simulink model "traj"  (R2020b)
settings: Solver=VariableStepAuto  StartTime=0.0  StopTime=All_Sim_time  MaxStep=0.05  RelTol=1e-3
model workspace (MAT data in the model file):
  Delay = 1
undefined symbols (not defined in the file or in its folder): All_Delay_betwn_actns, All_Maneuver_smoothness, Maneuver1_aggression, Maneuver2_aggression, Maneuver3_aggression, Maneuver4_aggression, Maneuver5_aggression
settings Model: Creator=pyoty  LastModifiedBy=liors

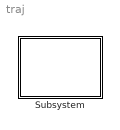
== system traj ==
  Subsystem : Subsystem

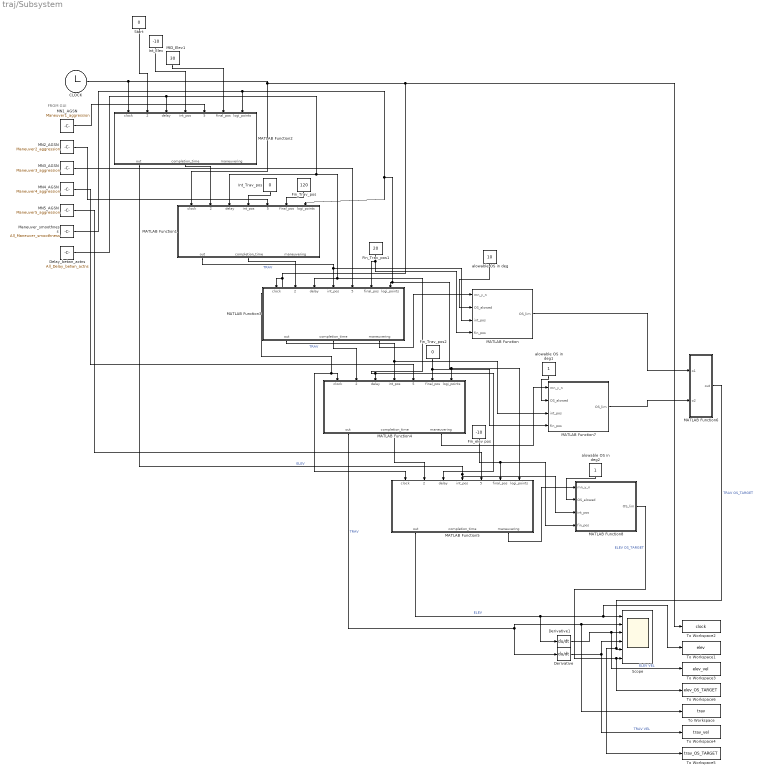
== system traj/Subsystem ==
  note: FROM GUI
  CLOCK : Clock
  Delay_betwn_actns : Constant  Value=All_Delay_betwn_actns
  Derivative : Derivative
  Derivative1 : Derivative
  Fin_Trav_pos : Constant  Value=120
  Fin_Trav_pos1 : Constant  Value=20
  Fin_Trav_pos2 : Constant  Value=0
  Fin_elev pos : Constant  Value=-10
  Int_Elev : Constant  Value=-10
  Int_Trav_pos : Constant  Value=0
  MATLAB Function : MATLAB Function  TreatAsAtomicUnit=on
  MATLAB Function1 : MATLAB Function  TreatAsAtomicUnit=on
  MATLAB Function2 : MATLAB Function  TreatAsAtomicUnit=on
  MATLAB Function3 : MATLAB Function  TreatAsAtomicUnit=on
  MATLAB Function4 : MATLAB Function  TreatAsAtomicUnit=on
  MATLAB Function5 : MATLAB Function  TreatAsAtomicUnit=on
  MATLAB Function6 : MATLAB Function  TreatAsAtomicUnit=on
  MATLAB Function7 : MATLAB Function  TreatAsAtomicUnit=on
  MATLAB Function8 : MATLAB Function  TreatAsAtomicUnit=on
  MID_Elev1 : Constant  Value=30
  MN1_AGSN : Constant  Value=Maneuver1_aggression
  MN2_AGSN : Constant  Value=Maneuver2_aggression
  MN3_AGSN : Constant  Value=Maneuver3_aggression
  MN4_AGSN : Constant  Value=Maneuver4_aggression
  MN5_AGSN : Constant  Value=Maneuver5_aggression
  Maneuver_smoothness : Constant  Value=All_Maneuver_smoothness
  Scope : Scope  NumInputPorts=6
  Start : Constant  Value=0
  To Workspace : ToWorkspace  VariableName=trav  SaveFormat=Timeseries  SampleTime=-1
  To Workspace1 : ToWorkspace  VariableName=elev  SaveFormat=Timeseries  SampleTime=-1
  To Workspace2 : ToWorkspace  VariableName=clock  SaveFormat=Timeseries  SampleTime=-1
  To Workspace3 : ToWorkspace  VariableName=elev_vel  SaveFormat=Timeseries  SampleTime=-1
  To Workspace4 : ToWorkspace  VariableName=trav_vel  SaveFormat=Timeseries  SampleTime=-1
  To Workspace5 : ToWorkspace  VariableName=trav_OS_TARGET  SaveFormat=Timeseries  SampleTime=-1
  To Workspace6 : ToWorkspace  VariableName=elev_OS_TARGET  SaveFormat=Timeseries  SampleTime=-1
  alowable OS in deg : Constant  Value=10
  alowable OS in deg1 : Constant
  alowable OS in deg2 : Constant
  wires:
  Derivative1/1 -> To Workspace3/1, Scope/3  "ELEV VEL"
  CLOCK/1 -> To Workspace2/1, MATLAB Function4/1(clock), MATLAB Function5/1(clock), MATLAB Function3/1(clock), MATLAB Function1/1(clock), MATLAB Function2/1(clock)
  MATLAB Function3/3(maneuvering) -> MATLAB Function/1(mn_y_n)
  Fin_elev pos/1 -> MATLAB Function8/4(fin_pos), MATLAB Function5/6(final_pos)
  MATLAB Function2/1(out) -> MATLAB Function8/3(int_pos), MATLAB Function5/4(int_pos)  "ELEV"
  Maneuver_smoothness/1 -> MATLAB Function4/7(logi_points), MATLAB Function5/7(logi_points), MATLAB Function3/7(logi_points), MATLAB Function1/7(logi_points), MATLAB Function2/7(logi_points)
  Int_Elev/1 -> MATLAB Function2/4(int_pos)
  Derivative/1 -> Scope/4, To Workspace4/1  "TRAV VEL"
  Start/1 -> MATLAB Function2/2(pev_mn_fin_time)
  MATLAB Function7/1(OS_lim) -> MATLAB Function6/2(o2)
  MN2_AGSN/1 -> MATLAB Function1/5(agressivness)
  MATLAB Function5/1(out) -> To Workspace1/1, Scope/1, Derivative1/1  "ELEV"
  MATLAB Function3/1(out) -> MATLAB Function7/3(int_pos), MATLAB Function4/4(int_pos)  "TRAV"
  alowable OS in deg1/1 -> MATLAB Function7/2(OS_alowed)
  Fin_Trav_pos1/1 -> MATLAB Function/4(fin_pos), MATLAB Function3/6(final_pos)
  MN5_AGSN/1 -> MATLAB Function5/5(agressivness)
  MATLAB Function1/1(out) -> MATLAB Function/3(int_pos), MATLAB Function3/4(int_pos)  "TRAV"
  Delay_betwn_actns/1 -> MATLAB Function5/3(delay), MATLAB Function4/3(delay), MATLAB Function3/3(delay), MATLAB Function1/3(delay), MATLAB Function2/3(delay)
  MN4_AGSN/1 -> MATLAB Function4/5(agressivness)
  MN1_AGSN/1 -> MATLAB Function2/5(agressivness)
  Int_Trav_pos/1 -> MATLAB Function1/4(int_pos)
  MATLAB Function3/2(completion_time) -> MATLAB Function4/2(pev_mn_fin_time)
  Fin_Trav_pos2/1 -> MATLAB Function7/4(fin_pos), MATLAB Function4/6(final_pos)
  alowable OS in deg/1 -> MATLAB Function/2(OS_alowed)
  MATLAB Function1/2(completion_time) -> MATLAB Function3/2(pev_mn_fin_time)
  MATLAB Function5/3(maneuvering) -> MATLAB Function8/1(mn_y_n)
  MATLAB Function2/2(completion_time) -> MATLAB Function1/2(pev_mn_fin_time)
  MN3_AGSN/1 -> MATLAB Function3/5(agressivness)
  Fin_Trav_pos/1 -> MATLAB Function1/6(final_pos)
  MID_Elev1/1 -> MATLAB Function2/6(final_pos)
  MATLAB Function4/1(out) -> Derivative/1, To Workspace/1, Scope/2  "TRAV"
  MATLAB Function6/1(out) -> To Workspace5/1, Scope/5  "TRAV OS_TARGET"
  MATLAB Function8/1(OS_lim) -> To Workspace6/1, Scope/6  "ELEV OS_TARGET"
  alowable OS in deg2/1 -> MATLAB Function8/2(OS_alowed)
  MATLAB Function/1(OS_lim) -> MATLAB Function6/1(o1)
  MATLAB Function4/3(maneuvering) -> MATLAB Function7/1(mn_y_n)
  MATLAB Function4/2(completion_time) -> MATLAB Function5/2(pev_mn_fin_time)

== matlab function traj/Subsystem/MATLAB Function ==
  data: mn_y_n input; OS_lim output; OS_alowed input; int_pos input; fin_pos input
function OS_lim = OS(mn_y_n,OS_alowed,int_pos,fin_pos)
if fin_pos>int_pos
    direction=1
else
    direction=-1
end

OS_lim = mn_y_n*(fin_pos+OS_alowed*direction);
if OS_lim==-inf
   OS_lim=inf
end
end

== matlab function traj/Subsystem/MATLAB Function6 ==
  data: o1 input; out output; o2 input
function out= min(o1,o2)
out=min([o1,o2])
end

== matlab function traj/Subsystem/MATLAB Function7 ==
  data: mn_y_n input; OS_lim output; OS_alowed input; int_pos input; fin_pos input
function OS_lim = OS(mn_y_n,OS_alowed,int_pos,fin_pos)
if fin_pos>int_pos
    direction=1
else
    direction=-1
end

OS_lim = mn_y_n*(fin_pos+OS_alowed*direction);
if OS_lim==-inf
   OS_lim=inf
end
end

== matlab function traj/Subsystem/MATLAB Function8 ==
  data: mn_y_n input; OS_lim output; OS_alowed input; int_pos input; fin_pos input
function OS_lim = OS(mn_y_n,OS_alowed,int_pos,fin_pos)
if fin_pos>int_pos
    direction=1
else
    direction=-1
end

OS_lim = mn_y_n*(fin_pos+OS_alowed*direction);
if OS_lim==-inf
   OS_lim=inf
end
end

== matlab function traj/Subsystem/MATLAB Function1 ==
  data: clock input; pev_mn_fin_time input; delay input; int_pos input; agressivness input; final_pos input; out output; completion_time output; logi_points input; maneuvering output
function [out,completion_time,maneuvering] =maneuver(clock,pev_mn_fin_time,delay,int_pos,agressivness,final_pos,logi_points)

if final_pos>int_pos
    direction=1
else
    direction=-1
end

slope=direction*agressivness
maneuvering=inf
mn_start_time=delay+pev_mn_fin_time
mn_completion_time=(final_pos-int_pos)/slope
completion_time=mn_completion_time+mn_start_time
coarsness=mn_completion_time/(logi_points+1)
mn_clock=clock-mn_start_time
coarse_clock=coarsness*floor(mn_clock/coarsness)
mn_clock2=clock+coarsness-mn_start_time
coarse_clock2=coarsness*floor(mn_clock2/coarsness)



if mn_clock<0
    out=int_pos
elseif clock<completion_time && mn_clock>=0
    adjust=mn_completion_time/18
    out1=((slope*mn_completion_time)/(1+exp((mn_completion_time/2-coarse_clock)/adjust)))    +int_pos
    out2=((slope*mn_completion_time)/(1+exp((mn_completion_time/2-coarse_clock2)/adjust)))    +int_pos
    sawtooth=mn_clock-coarse_clock
    new_slope=(out2-out1)/(coarsness)
    out=new_slope*sawtooth+out1
else
    out=final_pos
end

if mn_clock>=mn_completion_time/2
    maneuvering=1
end

if clock>=completion_time+delay+5/mn_completion_time
         maneuvering=inf
end
end

== matlab function traj/Subsystem/MATLAB Function3 ==
  data: clock input; pev_mn_fin_time input; delay input; int_pos input; agressivness input; final_pos input; out output; completion_time output; logi_points input; maneuvering output
function [out,completion_time,maneuvering] =maneuver(clock,pev_mn_fin_time,delay,int_pos,agressivness,final_pos,logi_points)

if final_pos>int_pos
    direction=1
else
    direction=-1
end

slope=direction*agressivness
maneuvering=inf
mn_start_time=delay+pev_mn_fin_time
mn_completion_time=(final_pos-int_pos)/slope
completion_time=mn_completion_time+mn_start_time
coarsness=mn_completion_time/(logi_points+1)
mn_clock=clock-mn_start_time
coarse_clock=coarsness*floor(mn_clock/coarsness)
mn_clock2=clock+coarsness-mn_start_time
coarse_clock2=coarsness*floor(mn_clock2/coarsness)



if mn_clock<0
    out=int_pos
elseif clock<completion_time && mn_clock>=0
    adjust=mn_completion_time/18
    out1=((slope*mn_completion_time)/(1+exp((mn_completion_time/2-coarse_clock)/adjust)))    +int_pos
    out2=((slope*mn_completion_time)/(1+exp((mn_completion_time/2-coarse_clock2)/adjust)))    +int_pos
    sawtooth=mn_clock-coarse_clock
    new_slope=(out2-out1)/(coarsness)
    out=new_slope*sawtooth+out1
else
    out=final_pos
end

if mn_clock>=mn_completion_time/2
    maneuvering=1
end

if clock>=completion_time+delay+5/mn_completion_time
         maneuvering=inf
end
end

== matlab function traj/Subsystem/MATLAB Function2 ==
  data: clock input; pev_mn_fin_time input; delay input; int_pos input; agressivness input; final_pos input; out output; completion_time output; logi_points input; maneuvering output
function [out,completion_time,maneuvering] =maneuver(clock,pev_mn_fin_time,delay,int_pos,agressivness,final_pos,logi_points)

if final_pos>int_pos
    direction=1
else
    direction=-1
end

slope=direction*agressivness
maneuvering=inf
mn_start_time=delay+pev_mn_fin_time
mn_completion_time=(final_pos-int_pos)/slope
completion_time=mn_completion_time+mn_start_time
coarsness=mn_completion_time/(logi_points+1)
mn_clock=clock-mn_start_time
coarse_clock=coarsness*floor(mn_clock/coarsness)
mn_clock2=clock+coarsness-mn_start_time
coarse_clock2=coarsness*floor(mn_clock2/coarsness)



if mn_clock<0
    out=int_pos
elseif clock<completion_time && mn_clock>=0
    adjust=mn_completion_time/18
    out1=((slope*mn_completion_time)/(1+exp((mn_completion_time/2-coarse_clock)/adjust)))    +int_pos
    out2=((slope*mn_completion_time)/(1+exp((mn_completion_time/2-coarse_clock2)/adjust)))    +int_pos
    sawtooth=mn_clock-coarse_clock
    new_slope=(out2-out1)/(coarsness)
    out=new_slope*sawtooth+out1
else
    out=final_pos
end

if mn_clock>=mn_completion_time/2
    maneuvering=1
end

if clock>=completion_time+delay+5/mn_completion_time
         maneuvering=inf
end
end

== matlab function traj/Subsystem/MATLAB Function4 ==
  data: clock input; pev_mn_fin_time input; delay input; int_pos input; agressivness input; final_pos input; out output; completion_time output; logi_points input; maneuvering output
function [out,completion_time,maneuvering] =maneuver(clock,pev_mn_fin_time,delay,int_pos,agressivness,final_pos,logi_points)

if final_pos>int_pos
    direction=1
else
    direction=-1
end

slope=direction*agressivness
maneuvering=inf
mn_start_time=delay+pev_mn_fin_time
mn_completion_time=(final_pos-int_pos)/slope
completion_time=mn_completion_time+mn_start_time
coarsness=mn_completion_time/(logi_points+1)
mn_clock=clock-mn_start_time
coarse_clock=coarsness*floor(mn_clock/coarsness)
mn_clock2=clock+coarsness-mn_start_time
coarse_clock2=coarsness*floor(mn_clock2/coarsness)



if mn_clock<0
    out=int_pos
elseif clock<completion_time && mn_clock>=0
    adjust=mn_completion_time/18
    out1=((slope*mn_completion_time)/(1+exp((mn_completion_time/2-coarse_clock)/adjust)))    +int_pos
    out2=((slope*mn_completion_time)/(1+exp((mn_completion_time/2-coarse_clock2)/adjust)))    +int_pos
    sawtooth=mn_clock-coarse_clock
    new_slope=(out2-out1)/(coarsness)
    out=new_slope*sawtooth+out1
else
    out=final_pos
end

if mn_clock>=mn_completion_time/2
    maneuvering=1
end

if clock>=completion_time+delay+5/mn_completion_time
         maneuvering=inf
end
end

== matlab function traj/Subsystem/MATLAB Function5 ==
  data: clock input; pev_mn_fin_time input; delay input; int_pos input; agressivness input; final_pos input; out output; completion_time output; logi_points input; maneuvering output
function [out,completion_time,maneuvering] =maneuver(clock,pev_mn_fin_time,delay,int_pos,agressivness,final_pos,logi_points)

if final_pos>int_pos
    direction=1
else
    direction=-1
end

slope=direction*agressivness
maneuvering=inf
mn_start_time=delay+pev_mn_fin_time
mn_completion_time=(final_pos-int_pos)/slope
completion_time=mn_completion_time+mn_start_time
coarsness=mn_completion_time/(logi_points+1)
mn_clock=clock-mn_start_time
coarse_clock=coarsness*floor(mn_clock/coarsness)
mn_clock2=clock+coarsness-mn_start_time
coarse_clock2=coarsness*floor(mn_clock2/coarsness)



if mn_clock<0
    out=int_pos
elseif clock<completion_time && mn_clock>=0
    adjust=mn_completion_time/18
    out1=((slope*mn_completion_time)/(1+exp((mn_completion_time/2-coarse_clock)/adjust)))    +int_pos
    out2=((slope*mn_completion_time)/(1+exp((mn_completion_time/2-coarse_clock2)/adjust)))    +int_pos
    sawtooth=mn_clock-coarse_clock
    new_slope=(out2-out1)/(coarsness)
    out=new_slope*sawtooth+out1
else
    out=final_pos
end

if mn_clock>=mn_completion_time/2
    maneuvering=1
end

if clock>=completion_time+delay+5/mn_completion_time
         maneuvering=inf
end
end
